simulink model "gm_UZ_EnDat_be4_segregation"  (R2023b)
settings: Solver=FixedStepAuto  StartTime=0  StopTime=0.000505  RelTol=1e-3
model workspace (MAT data in the model file):
  Select = 0
libraries: hdlsllib x74, simulink x21, hdlmdlgenlib x4, simulink_extras x1
(part 3 of 5)

== system gm_UZ_EnDat_be4_segregation/UZ_ENDAT/5timestorage/Compare To Constant ==
  u : Inport  OutDataTypeStr=fixdt(0,8,0,'DataTypeOverride', 'Off')  SampleTime=1e-08
  Compare : RelationalOperator  Operator===  OutDataTypeStr=boolean
  Constant : Constant  DisableCoverage=on  Value=const  OutDataTypeStr=Inherit: Inherit via back propagation  SampleTime=-1
  y : Outport  SampleTime=1e-08
  wires:
  u/1 -> Compare/1
  Compare/1 -> y/1
  Constant/1 -> Compare/2

== system gm_UZ_EnDat_be4_segregation/UZ_ENDAT/5timestorage/Compare To Constant1 ==
  u : Inport  OutDataTypeStr=fixdt(0,8,0,'DataTypeOverride', 'Off')  SampleTime=1e-08
  Compare : RelationalOperator  Operator===  OutDataTypeStr=boolean
  Constant : Constant  DisableCoverage=on  Value=const  OutDataTypeStr=Inherit: Inherit via back propagation  SampleTime=-1
  y : Outport  SampleTime=1e-08
  wires:
  u/1 -> Compare/1
  Compare/1 -> y/1
  Constant/1 -> Compare/2

== system gm_UZ_EnDat_be4_segregation/UZ_ENDAT/5timestorage/Compare To Constant2 ==
  u : Inport  OutDataTypeStr=fixdt(0,8,0,'DataTypeOverride', 'Off')  SampleTime=1e-08
  Compare : RelationalOperator  Operator===  OutDataTypeStr=boolean
  Constant : Constant  DisableCoverage=on  Value=const  OutDataTypeStr=Inherit: Inherit via back propagation  SampleTime=-1
  y : Outport  SampleTime=1e-08
  wires:
  u/1 -> Compare/1
  Compare/1 -> y/1
  Constant/1 -> Compare/2

== system gm_UZ_EnDat_be4_segregation/UZ_ENDAT/5timestorage/Compare To Constant3 ==
  u : Inport  OutDataTypeStr=fixdt(0,8,0,'DataTypeOverride', 'Off')  SampleTime=1e-08
  Compare : RelationalOperator  Operator===  OutDataTypeStr=boolean
  Constant : Constant  DisableCoverage=on  Value=const  OutDataTypeStr=Inherit: Inherit via back propagation  SampleTime=-1
  y : Outport  SampleTime=1e-08
  wires:
  u/1 -> Compare/1
  Compare/1 -> y/1
  Constant/1 -> Compare/2

== system gm_UZ_EnDat_be4_segregation/UZ_ENDAT/5timestorage/Compare To Constant4 ==
  u : Inport  OutDataTypeStr=fixdt(0,8,0,'DataTypeOverride', 'Off')  SampleTime=1e-08
  Compare : RelationalOperator  Operator===  OutDataTypeStr=boolean
  Constant : Constant  DisableCoverage=on  Value=const  OutDataTypeStr=Inherit: Inherit via back propagation  SampleTime=-1
  y : Outport  SampleTime=1e-08
  wires:
  u/1 -> Compare/1
  Compare/1 -> y/1
  Constant/1 -> Compare/2

== system gm_UZ_EnDat_be4_segregation/UZ_ENDAT/5timestorage/Storage20 ==
  Data : Inport  OutDataTypeStr=fixdt(0, 64, 0)  PortDimensions=1  SampleTime=1e-08
  Write : Inport  Port=2  OutDataTypeStr=boolean  PortDimensions=1  SampleTime=1e-08
  Compare To Zero : Subsystem  mask(Compare To Zero){relop===, OutDataTypeStr=boolean, ZeroCross=on}
      mask prompts: relop "Simulink:masks:Operator_MP"; OutDataTypeStr "Simulink:masks:OutputDataType_MP"; ZeroCross "Simulink:masks:EnableZerocrossingDetection_MP"
      mask help: Simulink:masks:CompareToZero_MD
      mask init:
      | OutDataTypeStr = 'boolean';
      | ZeroCross = 'on';
      | blkName = 'UZ_EnDat_be4_segregation/UZ_ENDAT/5timestorage/Storage20/Compare\nTo Zero';
      | relop = '==';
      | setValue = 'boolean';
      mask TypeOptions relop: == | ~= | < | <= | >= | >
      mask TypeOptions OutDataTypeStr: Simulink:masks:uint8 | Simulink:masks:boolean
      mask Callback ZeroCross: sl('zeroCrossEnable', gcbh);
      mask Display: disp([relop,' 0'])
  Logical Operator : Logic  Operator=NOT  Inputs=1  AllPortsSameDT=off  OutDataTypeStr=boolean  SampleTime=1e-08
  Logical Operator1 : Logic  Inputs=3  AllPortsSameDT=off  OutDataTypeStr=boolean  SampleTime=1e-08
  Logical Operator2 : Logic  Operator=NOT  Inputs=1  AllPortsSameDT=off  OutDataTypeStr=boolean  SampleTime=1e-08
  Relational Operator : RelationalOperator  Operator===  OutDataTypeStr=boolean  SampleTime=1e-08  InputSameDT=off
  Single Port RAM System : hdlsllib/HDL RAMs/Single Port RAM System  RAMType=Single port  AsyncRead=off  WriteOutputValue=Old data  RAMInitialValue=0  allowBusInputs=off  WritesHaveOutput=on  NumReads=0  NumWrites=1  SimulateUsing=Code generation
  adress : Constant  Value=20  OutDataTypeStr=uint8  SampleTime=1e-08
  t : Constant  Value=double(0)  OutDataTypeStr=boolean  SampleTime=1e-08
  out : Outport  SampleTime=1e-08
  wrok : Outport  Port=2  OutDataTypeStr=boolean  SampleTime=1e-08
  wires:
  Data/1 -> Compare To Zero/1(u), Relational Operator/2, Single Port RAM System/1
  Write/1 -> Logical Operator1/1
  Compare To Zero/1(y) -> Logical Operator2/1
  Logical Operator2/1 -> Logical Operator1/3
  t/1 -> wrok/1
  adress/1 -> Single Port RAM System/2
  Single Port RAM System/1 -> Relational Operator/1, out/1
  Relational Operator/1 -> Logical Operator/1
  Logical Operator/1 -> Logical Operator1/2
  Logical Operator1/1 -> Single Port RAM System/3

== system gm_UZ_EnDat_be4_segregation/UZ_ENDAT/5timestorage/Storage21 ==
  Data : Inport  OutDataTypeStr=fixdt(0, 64, 0)  PortDimensions=1  SampleTime=1e-08
  Write : Inport  Port=2  OutDataTypeStr=boolean  PortDimensions=1  SampleTime=1e-08
  Compare To Zero : Subsystem  mask(Compare To Zero){relop===, OutDataTypeStr=boolean, ZeroCross=on}
      mask prompts: relop "Simulink:masks:Operator_MP"; OutDataTypeStr "Simulink:masks:OutputDataType_MP"; ZeroCross "Simulink:masks:EnableZerocrossingDetection_MP"
      mask help: Simulink:masks:CompareToZero_MD
      mask init:
      | OutDataTypeStr = 'boolean';
      | ZeroCross = 'on';
      | blkName = 'UZ_EnDat_be4_segregation/UZ_ENDAT/5timestorage/Storage21/Compare\nTo Zero';
      | relop = '==';
      | setValue = 'boolean';
      mask TypeOptions relop: == | ~= | < | <= | >= | >
      mask TypeOptions OutDataTypeStr: Simulink:masks:uint8 | Simulink:masks:boolean
      mask Callback ZeroCross: sl('zeroCrossEnable', gcbh);
      mask Display: disp([relop,' 0'])
  Logical Operator : Logic  Operator=NOT  Inputs=1  AllPortsSameDT=off  OutDataTypeStr=boolean  SampleTime=1e-08
  Logical Operator1 : Logic  Inputs=3  AllPortsSameDT=off  OutDataTypeStr=boolean  SampleTime=1e-08
  Logical Operator2 : Logic  Operator=NOT  Inputs=1  AllPortsSameDT=off  OutDataTypeStr=boolean  SampleTime=1e-08
  Relational Operator : RelationalOperator  Operator===  OutDataTypeStr=boolean  SampleTime=1e-08  InputSameDT=off
  Single Port RAM System : hdlsllib/HDL RAMs/Single Port RAM System  RAMType=Single port  AsyncRead=off  WriteOutputValue=Old data  RAMInitialValue=0  allowBusInputs=off  WritesHaveOutput=on  NumReads=0  NumWrites=1  SimulateUsing=Code generation
  adress : Constant  Value=21  OutDataTypeStr=uint8  SampleTime=1e-08
  t : Constant  Value=double(0)  OutDataTypeStr=boolean  SampleTime=1e-08
  out : Outport  SampleTime=1e-08
  wrok : Outport  Port=2  OutDataTypeStr=boolean  SampleTime=1e-08
  wires:
  Data/1 -> Compare To Zero/1(u), Relational Operator/2, Single Port RAM System/1
  Write/1 -> Logical Operator1/1
  Compare To Zero/1(y) -> Logical Operator2/1
  Logical Operator2/1 -> Logical Operator1/3
  t/1 -> wrok/1
  adress/1 -> Single Port RAM System/2
  Single Port RAM System/1 -> Relational Operator/1, out/1
  Relational Operator/1 -> Logical Operator/1
  Logical Operator/1 -> Logical Operator1/2
  Logical Operator1/1 -> Single Port RAM System/3

== system gm_UZ_EnDat_be4_segregation/UZ_ENDAT/5timestorage/Storage22 ==
  Data : Inport  OutDataTypeStr=fixdt(0, 64, 0)  PortDimensions=1  SampleTime=1e-08
  Write : Inport  Port=2  OutDataTypeStr=boolean  PortDimensions=1  SampleTime=1e-08
  Compare To Zero : Subsystem  mask(Compare To Zero){relop===, OutDataTypeStr=boolean, ZeroCross=on}
      mask prompts: relop "Simulink:masks:Operator_MP"; OutDataTypeStr "Simulink:masks:OutputDataType_MP"; ZeroCross "Simulink:masks:EnableZerocrossingDetection_MP"
      mask help: Simulink:masks:CompareToZero_MD
      mask init:
      | OutDataTypeStr = 'boolean';
      | ZeroCross = 'on';
      | blkName = 'UZ_EnDat_be4_segregation/UZ_ENDAT/5timestorage/Storage22/Compare\nTo Zero';
      | relop = '==';
      | setValue = 'boolean';
      mask TypeOptions relop: == | ~= | < | <= | >= | >
      mask TypeOptions OutDataTypeStr: Simulink:masks:uint8 | Simulink:masks:boolean
      mask Callback ZeroCross: sl('zeroCrossEnable', gcbh);
      mask Display: disp([relop,' 0'])
  Logical Operator : Logic  Operator=NOT  Inputs=1  AllPortsSameDT=off  OutDataTypeStr=boolean  SampleTime=1e-08
  Logical Operator1 : Logic  Inputs=3  AllPortsSameDT=off  OutDataTypeStr=boolean  SampleTime=1e-08
  Logical Operator2 : Logic  Operator=NOT  Inputs=1  AllPortsSameDT=off  OutDataTypeStr=boolean  SampleTime=1e-08
  Relational Operator : RelationalOperator  Operator===  OutDataTypeStr=boolean  SampleTime=1e-08  InputSameDT=off
  Single Port RAM System : hdlsllib/HDL RAMs/Single Port RAM System  RAMType=Single port  AsyncRead=off  WriteOutputValue=Old data  RAMInitialValue=0  allowBusInputs=off  WritesHaveOutput=on  NumReads=0  NumWrites=1  SimulateUsing=Code generation
  adress : Constant  Value=22  OutDataTypeStr=uint8  SampleTime=1e-08
  t : Constant  Value=double(0)  OutDataTypeStr=boolean  SampleTime=1e-08
  out : Outport  SampleTime=1e-08
  wrok : Outport  Port=2  OutDataTypeStr=boolean  SampleTime=1e-08
  wires:
  Data/1 -> Compare To Zero/1(u), Relational Operator/2, Single Port RAM System/1
  Write/1 -> Logical Operator1/1
  Compare To Zero/1(y) -> Logical Operator2/1
  Logical Operator2/1 -> Logical Operator1/3
  t/1 -> wrok/1
  adress/1 -> Single Port RAM System/2
  Single Port RAM System/1 -> Relational Operator/1, out/1
  Relational Operator/1 -> Logical Operator/1
  Logical Operator/1 -> Logical Operator1/2
  Logical Operator1/1 -> Single Port RAM System/3

== system gm_UZ_EnDat_be4_segregation/UZ_ENDAT/5timestorage/Storage23 ==
  Data : Inport  OutDataTypeStr=fixdt(0, 64, 0)  PortDimensions=1  SampleTime=1e-08
  Write : Inport  Port=2  OutDataTypeStr=boolean  PortDimensions=1  SampleTime=1e-08
  Compare To Zero : Subsystem  mask(Compare To Zero){relop===, OutDataTypeStr=boolean, ZeroCross=on}
      mask prompts: relop "Simulink:masks:Operator_MP"; OutDataTypeStr "Simulink:masks:OutputDataType_MP"; ZeroCross "Simulink:masks:EnableZerocrossingDetection_MP"
      mask help: Simulink:masks:CompareToZero_MD
      mask init:
      | OutDataTypeStr = 'boolean';
      | ZeroCross = 'on';
      | blkName = 'UZ_EnDat_be4_segregation/UZ_ENDAT/5timestorage/Storage23/Compare\nTo Zero';
      | relop = '==';
      | setValue = 'boolean';
      mask TypeOptions relop: == | ~= | < | <= | >= | >
      mask TypeOptions OutDataTypeStr: Simulink:masks:uint8 | Simulink:masks:boolean
      mask Callback ZeroCross: sl('zeroCrossEnable', gcbh);
      mask Display: disp([relop,' 0'])
  Logical Operator : Logic  Operator=NOT  Inputs=1  AllPortsSameDT=off  OutDataTypeStr=boolean  SampleTime=1e-08
  Logical Operator1 : Logic  Inputs=3  AllPortsSameDT=off  OutDataTypeStr=boolean  SampleTime=1e-08
  Logical Operator2 : Logic  Operator=NOT  Inputs=1  AllPortsSameDT=off  OutDataTypeStr=boolean  SampleTime=1e-08
  Relational Operator : RelationalOperator  Operator===  OutDataTypeStr=boolean  SampleTime=1e-08  InputSameDT=off
  Single Port RAM System : hdlsllib/HDL RAMs/Single Port RAM System  RAMType=Single port  AsyncRead=off  WriteOutputValue=Old data  RAMInitialValue=0  allowBusInputs=off  WritesHaveOutput=on  NumReads=0  NumWrites=1  SimulateUsing=Code generation
  adress : Constant  Value=23  OutDataTypeStr=uint8  SampleTime=1e-08
  t : Constant  Value=double(0)  OutDataTypeStr=boolean  SampleTime=1e-08
  out : Outport  SampleTime=1e-08
  wrok : Outport  Port=2  OutDataTypeStr=boolean  SampleTime=1e-08
  wires:
  Data/1 -> Compare To Zero/1(u), Relational Operator/2, Single Port RAM System/1
  Write/1 -> Logical Operator1/1
  Compare To Zero/1(y) -> Logical Operator2/1
  Logical Operator2/1 -> Logical Operator1/3
  t/1 -> wrok/1
  adress/1 -> Single Port RAM System/2
  Single Port RAM System/1 -> Relational Operator/1, out/1
  Relational Operator/1 -> Logical Operator/1
  Logical Operator/1 -> Logical Operator1/2
  Logical Operator1/1 -> Single Port RAM System/3

== system gm_UZ_EnDat_be4_segregation/UZ_ENDAT/5timestorage/Storage24 ==
  Data : Inport  OutDataTypeStr=fixdt(0, 64, 0)  PortDimensions=1  SampleTime=1e-08
  Write : Inport  Port=2  OutDataTypeStr=boolean  PortDimensions=1  SampleTime=1e-08
  Compare To Zero : Subsystem  mask(Compare To Zero){relop===, OutDataTypeStr=boolean, ZeroCross=on}
      mask prompts: relop "Simulink:masks:Operator_MP"; OutDataTypeStr "Simulink:masks:OutputDataType_MP"; ZeroCross "Simulink:masks:EnableZerocrossingDetection_MP"
      mask help: Simulink:masks:CompareToZero_MD
      mask init:
      | OutDataTypeStr = 'boolean';
      | ZeroCross = 'on';
      | blkName = 'UZ_EnDat_be4_segregation/UZ_ENDAT/5timestorage/Storage24/Compare\nTo Zero';
      | relop = '==';
      | setValue = 'boolean';
      mask TypeOptions relop: == | ~= | < | <= | >= | >
      mask TypeOptions OutDataTypeStr: Simulink:masks:uint8 | Simulink:masks:boolean
      mask Callback ZeroCross: sl('zeroCrossEnable', gcbh);
      mask Display: disp([relop,' 0'])
  Logical Operator : Logic  Operator=NOT  Inputs=1  AllPortsSameDT=off  OutDataTypeStr=boolean  SampleTime=1e-08
  Logical Operator1 : Logic  Inputs=3  AllPortsSameDT=off  OutDataTypeStr=boolean  SampleTime=1e-08
  Logical Operator2 : Logic  Operator=NOT  Inputs=1  AllPortsSameDT=off  OutDataTypeStr=boolean  SampleTime=1e-08
  Relational Operator : RelationalOperator  Operator===  OutDataTypeStr=boolean  SampleTime=1e-08  InputSameDT=off
  Single Port RAM System : hdlsllib/HDL RAMs/Single Port RAM System  RAMType=Single port  AsyncRead=off  WriteOutputValue=Old data  RAMInitialValue=0  allowBusInputs=off  WritesHaveOutput=on  NumReads=0  NumWrites=1  SimulateUsing=Code generation
  adress : Constant  Value=24  OutDataTypeStr=uint8  SampleTime=1e-08
  t : Constant  Value=double(0)  OutDataTypeStr=boolean  SampleTime=1e-08
  out : Outport  SampleTime=1e-08
  wrok : Outport  Port=2  OutDataTypeStr=boolean  SampleTime=1e-08
  wires:
  Data/1 -> Compare To Zero/1(u), Relational Operator/2, Single Port RAM System/1
  Write/1 -> Logical Operator1/1
  Compare To Zero/1(y) -> Logical Operator2/1
  Logical Operator2/1 -> Logical Operator1/3
  t/1 -> wrok/1
  adress/1 -> Single Port RAM System/2
  Single Port RAM System/1 -> Relational Operator/1, out/1
  Relational Operator/1 -> Logical Operator/1
  Logical Operator/1 -> Logical Operator1/2
  Logical Operator1/1 -> Single Port RAM System/3

== system gm_UZ_EnDat_be4_segregation/UZ_ENDAT/5timestorage/Triggered Subsystem ==
  Trigger : Inport  OutDataTypeStr=boolean  SampleTime=1e-08
  Counter Limited : Subsystem  mask(Counter Limited){uplimit=double(4), tsamp=double(-1)}
      mask prompts: uplimit "Simulink:masks:UpperLimit_MP"; tsamp "Simulink:masks:SampleTime_MP"
      mask help: Simulink:masks:CounterLimited_MD
  Trigger_delay : Delay  DelayLength=double(1)  InitialCondition=0
  Trigger_delay_Initial_Val : Constant  OutDataTypeStr=boolean  SampleTime=1e-08
  Trigger_delay_ctrl_const : Constant  OutDataTypeStr=boolean  SampleTime=1e-08
  Trigger_delay_ctrl_delay : Delay  DelayLength=double(1)  InitialCondition=0
  Trigger_delay_switch : Switch  Criteria=u2 ~= 0  Threshold=double(0)  OutDataTypeStr=boolean  SampleTime=1e-08  SaturateOnIntegerOverflow=off  InputSameDT=off
  Trigger_delayed_inverted_and_Trigger : Logic  AllPortsSameDT=off  OutDataTypeStr=boolean  SampleTime=1e-08
  delayMatch : Delay  DelayLength=double(2)  InitialCondition=0
  not_Trigger_delayed : Logic  Operator=NOT  Inputs=1  AllPortsSameDT=off  OutDataTypeStr=boolean  SampleTime=1e-08
  Out1 : Outport  SampleTime=1e-08  InitialOutput=0
  wires:
  Trigger/1 -> Trigger_delayed_inverted_and_Trigger/2, Trigger_delay/1
  Counter Limited/1(y) -> Out1/1
  Trigger_delay_switch/1 -> not_Trigger_delayed/1
  not_Trigger_delayed/1 -> Trigger_delayed_inverted_and_Trigger/1
  Trigger_delayed_inverted_and_Trigger/1 -> Counter Limited/1(Trigger_emulated)
  Trigger_delay/1 -> Trigger_delay_switch/1
  Trigger_delay_Initial_Val/1 -> Trigger_delay_switch/3
  Trigger_delay_ctrl_const/1 -> Trigger_delay_ctrl_delay/1
  delayMatch/1 -> Trigger_delay_switch/2
  Trigger_delay_ctrl_delay/1 -> delayMatch/1

== system gm_UZ_EnDat_be4_segregation/UZ_ENDAT/CLKCNTER_ACT/Positional_Counter ==
  valueout : Inport  OutDataTypeStr=uint32  PortDimensions=1  SampleTime=1e-08
  Trigger : Inport  Port=2  OutDataTypeStr=boolean  SampleTime=1e-08
  Increment Stored Integer : Subsystem  mask(Stored Integer Value Increment){}
      mask help: Simulink:masks:StoredIntegerValueIncrement_MD
      mask Display: disp('Q++')
  Increment Stored Integer_out1bypassMux : MultiPortSwitch  DataPortOrder=Zero-based contiguous  Inputs=2  zeroidx=on  OutDataTypeStr=uint32  SampleTime=1e-08  SaturateOnIntegerOverflow=off  InputSameDT=off
  Trigger_delay : Delay  DelayLength=double(1)  InitialCondition=0
  Trigger_delayed_inverted_and_Trigger : Logic  AllPortsSameDT=off  OutDataTypeStr=boolean  SampleTime=1e-08
  not_Trigger_delayed : Logic  Operator=NOT  Inputs=1  AllPortsSameDT=off  OutDataTypeStr=boolean  SampleTime=1e-08
  out0_bypass : UnitDelay  InitialCondition="fi(0,0,32,0,\"hex\",\"00000000\")"  SampleTime=1e-08
  divider : Outport  SampleTime=1e-08  InitialOutput=0
  wires:
  Increment Stored Integer/1(y) -> Increment Stored Integer_out1bypassMux/3
  out0_bypass/1 -> Increment Stored Integer_out1bypassMux/2
  Trigger_delayed_inverted_and_Trigger/1 -> Increment Stored Integer_out1bypassMux/1
  not_Trigger_delayed/1 -> Trigger_delayed_inverted_and_Trigger/1
  Trigger_delay/1 -> not_Trigger_delayed/1
  Increment Stored Integer_out1bypassMux/1 -> out0_bypass/1, divider/1
  valueout/1 -> Increment Stored Integer/1(u)
  Trigger/1 -> Trigger_delay/1, Trigger_delayed_inverted_and_Trigger/2

== system gm_UZ_EnDat_be4_segregation/UZ_ENDAT/CLKCNTER_ACT/SetZero32 ==
  valin : Inport  OutDataTypeStr=uint32  PortDimensions=1  SampleTime=1e-08
  setzero : Inport  Port=2  OutDataTypeStr=boolean  PortDimensions=1  SampleTime=1e-08
  Trigger : Inport  Port=3  OutDataTypeStr=boolean  SampleTime=1e-08
  Constant1 : Constant  OutDataTypeStr=fixdt(0, 1, 0)  SampleTime=1e-08
  Constant2 : Constant  Value=0  OutDataTypeStr=fixdt(0, 1, 0)  SampleTime=1e-08
  Index Vector1 : MultiPortSwitch  DataPortOrder=Zero-based contiguous  Inputs=2  DiagnosticForDefault=None  zeroidx=on  OutDataTypeStr=fixdt(0, 1, 0)  SampleTime=1e-08  SaturateOnIntegerOverflow=off  InputSameDT=off
  Product : Product  Inputs=**  OutDataTypeStr=uint32  SaturateOnIntegerOverflow=on  SampleTime=1e-08
  Product_out1bypassMux : MultiPortSwitch  DataPortOrder=Zero-based contiguous  Inputs=2  zeroidx=on  OutDataTypeStr=uint32  SampleTime=1e-08  SaturateOnIntegerOverflow=off  InputSameDT=off
  Trigger_delay : Delay  DelayLength=double(1)  InitialCondition=0
  Trigger_delay_Initial_Val : Constant  OutDataTypeStr=boolean  SampleTime=1e-08
  Trigger_delay_ctrl_const : Constant  OutDataTypeStr=boolean  SampleTime=1e-08
  Trigger_delay_ctrl_delay : Delay  DelayLength=double(1)  InitialCondition=0
  Trigger_delay_switch : Switch  Criteria=u2 ~= 0  Threshold=double(0)  OutDataTypeStr=boolean  SampleTime=1e-08  SaturateOnIntegerOverflow=off  InputSameDT=off
  Trigger_delayed_inverted_and_Trigger : Logic  AllPortsSameDT=off  OutDataTypeStr=boolean  SampleTime=1e-08
  delayMatch{,1..5} (6 alike) : Delay  DelayLength=double(2)  InitialCondition=0
  not_Trigger_delayed : Logic  Operator=NOT  Inputs=1  AllPortsSameDT=off  OutDataTypeStr=boolean  SampleTime=1e-08
  out0_bypass : UnitDelay  InitialCondition=double(0)  SampleTime=1e-08
  out0_bypass_Initial_Val : Constant  OutDataTypeStr=uint32  SampleTime=1e-08
  out0_bypass_ctrl_const : Constant  OutDataTypeStr=boolean  SampleTime=1e-08
  out0_bypass_ctrl_delay : Delay  DelayLength=double(1)  InitialCondition=0
  out0_bypass_switch : Switch  Criteria=u2 ~= 0  Threshold=double(0)  OutDataTypeStr=uint32  SampleTime=1e-08  SaturateOnIntegerOverflow=off  InputSameDT=off
  valueout : Outport  SampleTime=1e-08  InitialOutput=0  VectorParamsAs1DForOutWhenUnconnected=off
  wires:
  Trigger/1 -> Trigger_delayed_inverted_and_Trigger/2, Trigger_delay/1
  valin/1 -> Product/2
  setzero/1 -> Index Vector1/1
  Trigger_delay_switch/1 -> not_Trigger_delayed/1
  not_Trigger_delayed/1 -> Trigger_delayed_inverted_and_Trigger/1
  Trigger_delay/1 -> Trigger_delay_switch/1
  delayMatch1/1 -> Trigger_delay_switch/3
  delayMatch/1 -> Trigger_delay_switch/2
  Index Vector1/1 -> Product/1
  delayMatch2/1 -> Index Vector1/2
  delayMatch3/1 -> Index Vector1/3
  Trigger_delay_ctrl_delay/1 -> delayMatch/1
  Trigger_delay_Initial_Val/1 -> delayMatch1/1
  Constant1/1 -> delayMatch2/1
  Constant2/1 -> delayMatch3/1
  out0_bypass_ctrl_delay/1 -> delayMatch4/1
  out0_bypass_Initial_Val/1 -> delayMatch5/1
  Product_out1bypassMux/1 -> out0_bypass/1, valueout/1
  out0_bypass/1 -> out0_bypass_switch/1
  delayMatch4/1 -> out0_bypass_switch/2
  delayMatch5/1 -> out0_bypass_switch/3
  Trigger_delayed_inverted_and_Trigger/1 -> Product_out1bypassMux/1
  Product/1 -> Product_out1bypassMux/3
  out0_bypass_switch/1 -> Product_out1bypassMux/2
  out0_bypass_ctrl_const/1 -> out0_bypass_ctrl_delay/1
  Trigger_delay_ctrl_const/1 -> Trigger_delay_ctrl_delay/1

== system gm_UZ_EnDat_be4_segregation/UZ_ENDAT/CLKCNTER_RAMPUP/Positional_Counter ==
  valueout : Inport  OutDataTypeStr=uint32  PortDimensions=1  SampleTime=1e-08
  Trigger : Inport  Port=2  OutDataTypeStr=boolean  SampleTime=1e-08
  Increment Stored Integer : Subsystem  mask(Stored Integer Value Increment){}
      mask help: Simulink:masks:StoredIntegerValueIncrement_MD
      mask Display: disp('Q++')
  Increment Stored Integer_out1bypassMux : MultiPortSwitch  DataPortOrder=Zero-based contiguous  Inputs=2  zeroidx=on  OutDataTypeStr=uint32  SampleTime=1e-08  SaturateOnIntegerOverflow=off  InputSameDT=off
  Trigger_delay : Delay  DelayLength=double(1)  InitialCondition=0
  Trigger_delayed_inverted_and_Trigger : Logic  AllPortsSameDT=off  OutDataTypeStr=boolean  SampleTime=1e-08
  not_Trigger_delayed : Logic  Operator=NOT  Inputs=1  AllPortsSameDT=off  OutDataTypeStr=boolean  SampleTime=1e-08
  out0_bypass : UnitDelay  InitialCondition="fi(0,0,32,0,\"hex\",\"00000000\")"  SampleTime=1e-08
  divider : Outport  SampleTime=1e-08  InitialOutput=0
  wires:
  Increment Stored Integer/1(y) -> Increment Stored Integer_out1bypassMux/3
  out0_bypass/1 -> Increment Stored Integer_out1bypassMux/2
  Trigger_delayed_inverted_and_Trigger/1 -> Increment Stored Integer_out1bypassMux/1
  not_Trigger_delayed/1 -> Trigger_delayed_inverted_and_Trigger/1
  Trigger_delay/1 -> not_Trigger_delayed/1
  Increment Stored Integer_out1bypassMux/1 -> out0_bypass/1, divider/1
  valueout/1 -> Increment Stored Integer/1(u)
  Trigger/1 -> Trigger_delay/1, Trigger_delayed_inverted_and_Trigger/2

== system gm_UZ_EnDat_be4_segregation/UZ_ENDAT/CLKCNTER_RAMPUP/SetZero32 ==
  valin : Inport  OutDataTypeStr=uint32  PortDimensions=1  SampleTime=1e-08
  setzero : Inport  Port=2  OutDataTypeStr=boolean  PortDimensions=1  SampleTime=1e-08
  Trigger : Inport  Port=3  OutDataTypeStr=boolean  SampleTime=1e-08
  Constant1 : Constant  OutDataTypeStr=fixdt(0, 1, 0)  SampleTime=1e-08
  Constant2 : Constant  Value=0  OutDataTypeStr=fixdt(0, 1, 0)  SampleTime=1e-08
  Index Vector1 : MultiPortSwitch  DataPortOrder=Zero-based contiguous  Inputs=2  DiagnosticForDefault=None  zeroidx=on  OutDataTypeStr=fixdt(0, 1, 0)  SampleTime=1e-08  SaturateOnIntegerOverflow=off  InputSameDT=off
  Product : Product  Inputs=**  OutDataTypeStr=uint32  SaturateOnIntegerOverflow=on  SampleTime=1e-08
  Product_out1bypassMux : MultiPortSwitch  DataPortOrder=Zero-based contiguous  Inputs=2  zeroidx=on  OutDataTypeStr=uint32  SampleTime=1e-08  SaturateOnIntegerOverflow=off  InputSameDT=off
  Trigger_delay : Delay  DelayLength=double(1)  InitialCondition=0
  Trigger_delay_Initial_Val : Constant  OutDataTypeStr=boolean  SampleTime=1e-08
  Trigger_delay_ctrl_const : Constant  OutDataTypeStr=boolean  SampleTime=1e-08
  Trigger_delay_ctrl_delay : Delay  DelayLength=double(1)  InitialCondition=0
  Trigger_delay_switch : Switch  Criteria=u2 ~= 0  Threshold=double(0)  OutDataTypeStr=boolean  SampleTime=1e-08  SaturateOnIntegerOverflow=off  InputSameDT=off
  Trigger_delayed_inverted_and_Trigger : Logic  AllPortsSameDT=off  OutDataTypeStr=boolean  SampleTime=1e-08
  not_Trigger_delayed : Logic  Operator=NOT  Inputs=1  AllPortsSameDT=off  OutDataTypeStr=boolean  SampleTime=1e-08
  out0_bypass : UnitDelay  InitialCondition=double(0)  SampleTime=1e-08
  out0_bypass_Initial_Val : Constant  OutDataTypeStr=uint32  SampleTime=1e-08
  out0_bypass_ctrl_const : Constant  OutDataTypeStr=boolean  SampleTime=1e-08
  out0_bypass_ctrl_delay : Delay  DelayLength=double(1)  InitialCondition=0
  out0_bypass_switch : Switch  Criteria=u2 ~= 0  Threshold=double(0)  OutDataTypeStr=uint32  SampleTime=1e-08  SaturateOnIntegerOverflow=off  InputSameDT=off
  valueout : Outport  SampleTime=1e-08  InitialOutput=0  VectorParamsAs1DForOutWhenUnconnected=off
  wires:
  Trigger/1 -> Trigger_delayed_inverted_and_Trigger/2, Trigger_delay/1
  valin/1 -> Product/2
  setzero/1 -> Index Vector1/1
  Product_out1bypassMux/1 -> valueout/1, out0_bypass/1
  Trigger_delay_switch/1 -> not_Trigger_delayed/1
  not_Trigger_delayed/1 -> Trigger_delayed_inverted_and_Trigger/1
  Trigger_delay/1 -> Trigger_delay_switch/1
  Trigger_delay_Initial_Val/1 -> Trigger_delay_switch/3
  Trigger_delay_ctrl_delay/1 -> Trigger_delay_switch/2
  Index Vector1/1 -> Product/1
  Constant1/1 -> Index Vector1/2
  Constant2/1 -> Index Vector1/3
  out0_bypass/1 -> out0_bypass_switch/1
  out0_bypass_ctrl_delay/1 -> out0_bypass_switch/2
  out0_bypass_Initial_Val/1 -> out0_bypass_switch/3
  Trigger_delayed_inverted_and_Trigger/1 -> Product_out1bypassMux/1
  Product/1 -> Product_out1bypassMux/3
  out0_bypass_switch/1 -> Product_out1bypassMux/2
  out0_bypass_ctrl_const/1 -> out0_bypass_ctrl_delay/1
  Trigger_delay_ctrl_const/1 -> Trigger_delay_ctrl_delay/1

== system gm_UZ_EnDat_be4_segregation/UZ_ENDAT/CLKDIV1/Triggered Subsystem ==
  D : Inport  OutDataTypeStr=boolean  PortDimensions=1  SampleTime=1e-08
  Trigger : Inport  Port=2  OutDataTypeStr=boolean  SampleTime=1e-08
  DbypassMux : MultiPortSwitch  DataPortOrder=Zero-based contiguous  Inputs=2  zeroidx=on  SampleTime=1e-08  SaturateOnIntegerOverflow=off  InputSameDT=off
  Trigger_delay : Delay  DelayLength=double(1)  InitialCondition=0
  Trigger_delay_Initial_Val : Constant  OutDataTypeStr=boolean  SampleTime=1e-08
  Trigger_delay_ctrl_const : Constant  OutDataTypeStr=boolean  SampleTime=1e-08
  Trigger_delay_ctrl_delay : Delay  DelayLength=double(1)  InitialCondition=0
  Trigger_delay_switch : Switch  Criteria=u2 ~= 0  Threshold=double(0)  OutDataTypeStr=boolean  SampleTime=1e-08  SaturateOnIntegerOverflow=off  InputSameDT=off
  Trigger_delayed_inverted_and_Trigger : Logic  AllPortsSameDT=off  OutDataTypeStr=boolean  SampleTime=1e-08
  not_Trigger_delayed : Logic  Operator=NOT  Inputs=1  AllPortsSameDT=off  OutDataTypeStr=boolean  SampleTime=1e-08
  out0_bypass : UnitDelay  SampleTime=1e-08
  Q : Outport  SampleTime=1e-08  InitialOutput=0
  wires:
  Trigger/1 -> Trigger_delayed_inverted_and_Trigger/2, Trigger_delay/1
  DbypassMux/1 -> Q/1, out0_bypass/1
  Trigger_delay_switch/1 -> not_Trigger_delayed/1
  not_Trigger_delayed/1 -> Trigger_delayed_inverted_and_Trigger/1
  Trigger_delay/1 -> Trigger_delay_switch/1
  Trigger_delay_Initial_Val/1 -> Trigger_delay_switch/3
  Trigger_delay_ctrl_delay/1 -> Trigger_delay_switch/2
  Trigger_delayed_inverted_and_Trigger/1 -> DbypassMux/1
  out0_bypass/1 -> DbypassMux/2
  D/1 -> DbypassMux/3
  Trigger_delay_ctrl_const/1 -> Trigger_delay_ctrl_delay/1

== system gm_UZ_EnDat_be4_segregation/UZ_ENDAT/CLKDIV3/Triggered Subsystem ==
  D : Inport  OutDataTypeStr=boolean  PortDimensions=1  SampleTime=1e-08
  Trigger : Inport  Port=2  OutDataTypeStr=boolean  SampleTime=1e-08
  DbypassMux : MultiPortSwitch  DataPortOrder=Zero-based contiguous  Inputs=2  zeroidx=on  SampleTime=1e-08  SaturateOnIntegerOverflow=off  InputSameDT=off
  Trigger_delay : Delay  DelayLength=double(1)  InitialCondition=0
  Trigger_delay_Initial_Val : Constant  OutDataTypeStr=boolean  SampleTime=1e-08
  Trigger_delay_ctrl_const : Constant  OutDataTypeStr=boolean  SampleTime=1e-08
  Trigger_delay_ctrl_delay : Delay  DelayLength=double(1)  InitialCondition=0
  Trigger_delay_switch : Switch  Criteria=u2 ~= 0  Threshold=double(0)  OutDataTypeStr=boolean  SampleTime=1e-08  SaturateOnIntegerOverflow=off  InputSameDT=off
  Trigger_delayed_inverted_and_Trigger : Logic  AllPortsSameDT=off  OutDataTypeStr=boolean  SampleTime=1e-08
  not_Trigger_delayed : Logic  Operator=NOT  Inputs=1  AllPortsSameDT=off  OutDataTypeStr=boolean  SampleTime=1e-08
  out0_bypass : UnitDelay  SampleTime=1e-08
  Q : Outport  SampleTime=1e-08  InitialOutput=0
  wires:
  Trigger_delay_ctrl_const/1 -> Trigger_delay_ctrl_delay/1
  D/1 -> DbypassMux/3
  out0_bypass/1 -> DbypassMux/2
  Trigger_delayed_inverted_and_Trigger/1 -> DbypassMux/1
  Trigger_delay_ctrl_delay/1 -> Trigger_delay_switch/2
  Trigger_delay_Initial_Val/1 -> Trigger_delay_switch/3
  Trigger_delay/1 -> Trigger_delay_switch/1
  not_Trigger_delayed/1 -> Trigger_delayed_inverted_and_Trigger/1
  Trigger_delay_switch/1 -> not_Trigger_delayed/1
  DbypassMux/1 -> out0_bypass/1, Q/1
  Trigger/1 -> Trigger_delay/1, Trigger_delayed_inverted_and_Trigger/2

== system gm_UZ_EnDat_be4_segregation/UZ_ENDAT/CLKDIV4/Triggered Subsystem ==
  D : Inport  OutDataTypeStr=boolean  PortDimensions=1  SampleTime=1e-08
  Trigger : Inport  Port=2  OutDataTypeStr=boolean  SampleTime=1e-08
  DbypassMux : MultiPortSwitch  DataPortOrder=Zero-based contiguous  Inputs=2  zeroidx=on  SampleTime=1e-08  SaturateOnIntegerOverflow=off  InputSameDT=off
  Trigger_delay : Delay  DelayLength=double(1)  InitialCondition=0
  Trigger_delay_Initial_Val : Constant  OutDataTypeStr=boolean  SampleTime=1e-08
  Trigger_delay_ctrl_const : Constant  OutDataTypeStr=boolean  SampleTime=1e-08
  Trigger_delay_ctrl_delay : Delay  DelayLength=double(1)  InitialCondition=0
  Trigger_delay_switch : Switch  Criteria=u2 ~= 0  Threshold=double(0)  OutDataTypeStr=boolean  SampleTime=1e-08  SaturateOnIntegerOverflow=off  InputSameDT=off
  Trigger_delayed_inverted_and_Trigger : Logic  AllPortsSameDT=off  OutDataTypeStr=boolean  SampleTime=1e-08
  not_Trigger_delayed : Logic  Operator=NOT  Inputs=1  AllPortsSameDT=off  OutDataTypeStr=boolean  SampleTime=1e-08
  out0_bypass : UnitDelay  SampleTime=1e-08
  Q : Outport  SampleTime=1e-08  InitialOutput=0
  wires:
  Trigger_delay_ctrl_const/1 -> Trigger_delay_ctrl_delay/1
  D/1 -> DbypassMux/3
  out0_bypass/1 -> DbypassMux/2
  Trigger_delayed_inverted_and_Trigger/1 -> DbypassMux/1
  Trigger_delay_ctrl_delay/1 -> Trigger_delay_switch/2
  Trigger_delay_Initial_Val/1 -> Trigger_delay_switch/3
  Trigger_delay/1 -> Trigger_delay_switch/1
  not_Trigger_delayed/1 -> Trigger_delayed_inverted_and_Trigger/1
  Trigger_delay_switch/1 -> not_Trigger_delayed/1
  DbypassMux/1 -> out0_bypass/1, Q/1
  Trigger/1 -> Trigger_delay/1, Trigger_delayed_inverted_and_Trigger/2

== system gm_UZ_EnDat_be4_segregation/UZ_ENDAT/CLKDIV5/Triggered Subsystem ==
  D : Inport  OutDataTypeStr=boolean  PortDimensions=1  SampleTime=1e-08
  Trigger : Inport  Port=2  OutDataTypeStr=boolean  SampleTime=1e-08
  DbypassMux : MultiPortSwitch  DataPortOrder=Zero-based contiguous  Inputs=2  zeroidx=on  SampleTime=1e-08  SaturateOnIntegerOverflow=off  InputSameDT=off
  Trigger_delay : Delay  DelayLength=double(1)  InitialCondition=0
  Trigger_delay_Initial_Val : Constant  OutDataTypeStr=boolean  SampleTime=1e-08
  Trigger_delay_ctrl_const : Constant  OutDataTypeStr=boolean  SampleTime=1e-08
  Trigger_delay_ctrl_delay : Delay  DelayLength=double(1)  InitialCondition=0
  Trigger_delay_switch : Switch  Criteria=u2 ~= 0  Threshold=double(0)  OutDataTypeStr=boolean  SampleTime=1e-08  SaturateOnIntegerOverflow=off  InputSameDT=off
  Trigger_delayed_inverted_and_Trigger : Logic  AllPortsSameDT=off  OutDataTypeStr=boolean  SampleTime=1e-08
  not_Trigger_delayed : Logic  Operator=NOT  Inputs=1  AllPortsSameDT=off  OutDataTypeStr=boolean  SampleTime=1e-08
  out0_bypass : UnitDelay  SampleTime=1e-08
  Q : Outport  SampleTime=1e-08  InitialOutput=0
  wires:
  Trigger_delay_ctrl_const/1 -> Trigger_delay_ctrl_delay/1
  D/1 -> DbypassMux/3
  out0_bypass/1 -> DbypassMux/2
  Trigger_delayed_inverted_and_Trigger/1 -> DbypassMux/1
  Trigger_delay_ctrl_delay/1 -> Trigger_delay_switch/2
  Trigger_delay_Initial_Val/1 -> Trigger_delay_switch/3
  Trigger_delay/1 -> Trigger_delay_switch/1
  not_Trigger_delayed/1 -> Trigger_delayed_inverted_and_Trigger/1
  Trigger_delay_switch/1 -> not_Trigger_delayed/1
  DbypassMux/1 -> out0_bypass/1, Q/1
  Trigger/1 -> Trigger_delay/1, Trigger_delayed_inverted_and_Trigger/2

== system gm_UZ_EnDat_be4_segregation/UZ_ENDAT/CLKDIV6/Triggered Subsystem ==
  D : Inport  OutDataTypeStr=boolean  PortDimensions=1  SampleTime=1e-08
  Trigger : Inport  Port=2  OutDataTypeStr=boolean  SampleTime=1e-08
  DbypassMux : MultiPortSwitch  DataPortOrder=Zero-based contiguous  Inputs=2  zeroidx=on  SampleTime=1e-08  SaturateOnIntegerOverflow=off  InputSameDT=off
  Trigger_delay : Delay  DelayLength=double(1)  InitialCondition=0
  Trigger_delay_Initial_Val : Constant  OutDataTypeStr=boolean  SampleTime=1e-08
  Trigger_delay_ctrl_const : Constant  OutDataTypeStr=boolean  SampleTime=1e-08
  Trigger_delay_ctrl_delay : Delay  DelayLength=double(1)  InitialCondition=0
  Trigger_delay_switch : Switch  Criteria=u2 ~= 0  Threshold=double(0)  OutDataTypeStr=boolean  SampleTime=1e-08  SaturateOnIntegerOverflow=off  InputSameDT=off
  Trigger_delayed_inverted_and_Trigger : Logic  AllPortsSameDT=off  OutDataTypeStr=boolean  SampleTime=1e-08
  not_Trigger_delayed : Logic  Operator=NOT  Inputs=1  AllPortsSameDT=off  OutDataTypeStr=boolean  SampleTime=1e-08
  out0_bypass : UnitDelay  SampleTime=1e-08
  Q : Outport  SampleTime=1e-08  InitialOutput=0
  wires:
  Trigger_delay_ctrl_const/1 -> Trigger_delay_ctrl_delay/1
  D/1 -> DbypassMux/3
  out0_bypass/1 -> DbypassMux/2
  Trigger_delayed_inverted_and_Trigger/1 -> DbypassMux/1
  Trigger_delay_ctrl_delay/1 -> Trigger_delay_switch/2
  Trigger_delay_Initial_Val/1 -> Trigger_delay_switch/3
  Trigger_delay/1 -> Trigger_delay_switch/1
  not_Trigger_delayed/1 -> Trigger_delayed_inverted_and_Trigger/1
  Trigger_delay_switch/1 -> not_Trigger_delayed/1
  DbypassMux/1 -> out0_bypass/1, Q/1
  Trigger/1 -> Trigger_delay/1, Trigger_delayed_inverted_and_Trigger/2

== system gm_UZ_EnDat_be4_segregation/UZ_ENDAT/CLKDIV7/Triggered Subsystem ==
  D : Inport  OutDataTypeStr=boolean  PortDimensions=1  SampleTime=1e-08
  Trigger : Inport  Port=2  OutDataTypeStr=boolean  SampleTime=1e-08
  DbypassMux : MultiPortSwitch  DataPortOrder=Zero-based contiguous  Inputs=2  zeroidx=on  SampleTime=1e-08  SaturateOnIntegerOverflow=off  InputSameDT=off
  Trigger_delay : Delay  DelayLength=double(1)  InitialCondition=0
  Trigger_delay_Initial_Val : Constant  OutDataTypeStr=boolean  SampleTime=1e-08
  Trigger_delay_ctrl_const : Constant  OutDataTypeStr=boolean  SampleTime=1e-08
  Trigger_delay_ctrl_delay : Delay  DelayLength=double(1)  InitialCondition=0
  Trigger_delay_switch : Switch  Criteria=u2 ~= 0  Threshold=double(0)  OutDataTypeStr=boolean  SampleTime=1e-08  SaturateOnIntegerOverflow=off  InputSameDT=off
  Trigger_delayed_inverted_and_Trigger : Logic  AllPortsSameDT=off  OutDataTypeStr=boolean  SampleTime=1e-08
  not_Trigger_delayed : Logic  Operator=NOT  Inputs=1  AllPortsSameDT=off  OutDataTypeStr=boolean  SampleTime=1e-08
  out0_bypass : UnitDelay  SampleTime=1e-08
  Q : Outport  SampleTime=1e-08  InitialOutput=0
  wires:
  Trigger_delay_ctrl_const/1 -> Trigger_delay_ctrl_delay/1
  D/1 -> DbypassMux/3
  out0_bypass/1 -> DbypassMux/2
  Trigger_delayed_inverted_and_Trigger/1 -> DbypassMux/1
  Trigger_delay_ctrl_delay/1 -> Trigger_delay_switch/2
  Trigger_delay_Initial_Val/1 -> Trigger_delay_switch/3
  Trigger_delay/1 -> Trigger_delay_switch/1
  not_Trigger_delayed/1 -> Trigger_delayed_inverted_and_Trigger/1
  Trigger_delay_switch/1 -> not_Trigger_delayed/1
  DbypassMux/1 -> out0_bypass/1, Q/1
  Trigger/1 -> Trigger_delay/1, Trigger_delayed_inverted_and_Trigger/2

== system gm_UZ_EnDat_be4_segregation/UZ_ENDAT/CLKDIV8/Triggered Subsystem ==
  D : Inport  OutDataTypeStr=boolean  PortDimensions=1  SampleTime=1e-08
  Trigger : Inport  Port=2  OutDataTypeStr=boolean  SampleTime=1e-08
  DbypassMux : MultiPortSwitch  DataPortOrder=Zero-based contiguous  Inputs=2  zeroidx=on  SampleTime=1e-08  SaturateOnIntegerOverflow=off  InputSameDT=off
  Trigger_delay : Delay  DelayLength=double(1)  InitialCondition=0
  Trigger_delay_Initial_Val : Constant  OutDataTypeStr=boolean  SampleTime=1e-08
  Trigger_delay_ctrl_const : Constant  OutDataTypeStr=boolean  SampleTime=1e-08
  Trigger_delay_ctrl_delay : Delay  DelayLength=double(1)  InitialCondition=0
  Trigger_delay_switch : Switch  Criteria=u2 ~= 0  Threshold=double(0)  OutDataTypeStr=boolean  SampleTime=1e-08  SaturateOnIntegerOverflow=off  InputSameDT=off
  Trigger_delayed_inverted_and_Trigger : Logic  AllPortsSameDT=off  OutDataTypeStr=boolean  SampleTime=1e-08
  not_Trigger_delayed : Logic  Operator=NOT  Inputs=1  AllPortsSameDT=off  OutDataTypeStr=boolean  SampleTime=1e-08
  out0_bypass : UnitDelay  SampleTime=1e-08
  Q : Outport  SampleTime=1e-08  InitialOutput=0
  wires:
  Trigger_delay_ctrl_const/1 -> Trigger_delay_ctrl_delay/1
  D/1 -> DbypassMux/3
  out0_bypass/1 -> DbypassMux/2
  Trigger_delayed_inverted_and_Trigger/1 -> DbypassMux/1
  Trigger_delay_ctrl_delay/1 -> Trigger_delay_switch/2
  Trigger_delay_Initial_Val/1 -> Trigger_delay_switch/3
  Trigger_delay/1 -> Trigger_delay_switch/1
  not_Trigger_delayed/1 -> Trigger_delayed_inverted_and_Trigger/1
  Trigger_delay_switch/1 -> not_Trigger_delayed/1
  DbypassMux/1 -> out0_bypass/1, Q/1
  Trigger/1 -> Trigger_delay/1, Trigger_delayed_inverted_and_Trigger/2

== system gm_UZ_EnDat_be4_segregation/UZ_ENDAT/CLKDIV9/Triggered Subsystem ==
  D : Inport  OutDataTypeStr=boolean  PortDimensions=1  SampleTime=1e-08
  Trigger : Inport  Port=2  OutDataTypeStr=boolean  SampleTime=1e-08
  DbypassMux : MultiPortSwitch  DataPortOrder=Zero-based contiguous  Inputs=2  zeroidx=on  SampleTime=1e-08  SaturateOnIntegerOverflow=off  InputSameDT=off
  Trigger_delay : Delay  DelayLength=double(1)  InitialCondition=0
  Trigger_delay_Initial_Val : Constant  OutDataTypeStr=boolean  SampleTime=1e-08
  Trigger_delay_ctrl_const : Constant  OutDataTypeStr=boolean  SampleTime=1e-08
  Trigger_delay_ctrl_delay : Delay  DelayLength=double(1)  InitialCondition=0
  Trigger_delay_switch : Switch  Criteria=u2 ~= 0  Threshold=double(0)  OutDataTypeStr=boolean  SampleTime=1e-08  SaturateOnIntegerOverflow=off  InputSameDT=off
  Trigger_delayed_inverted_and_Trigger : Logic  AllPortsSameDT=off  OutDataTypeStr=boolean  SampleTime=1e-08
  not_Trigger_delayed : Logic  Operator=NOT  Inputs=1  AllPortsSameDT=off  OutDataTypeStr=boolean  SampleTime=1e-08
  out0_bypass : UnitDelay  SampleTime=1e-08
  Q : Outport  SampleTime=1e-08  InitialOutput=0
  wires:
  Trigger_delay_ctrl_const/1 -> Trigger_delay_ctrl_delay/1
  D/1 -> DbypassMux/3
  out0_bypass/1 -> DbypassMux/2
  Trigger_delayed_inverted_and_Trigger/1 -> DbypassMux/1
  Trigger_delay_ctrl_delay/1 -> Trigger_delay_switch/2
  Trigger_delay_Initial_Val/1 -> Trigger_delay_switch/3
  Trigger_delay/1 -> Trigger_delay_switch/1
  not_Trigger_delayed/1 -> Trigger_delayed_inverted_and_Trigger/1
  Trigger_delay_switch/1 -> not_Trigger_delayed/1
  DbypassMux/1 -> out0_bypass/1, Q/1
  Trigger/1 -> Trigger_delay/1, Trigger_delayed_inverted_and_Trigger/2

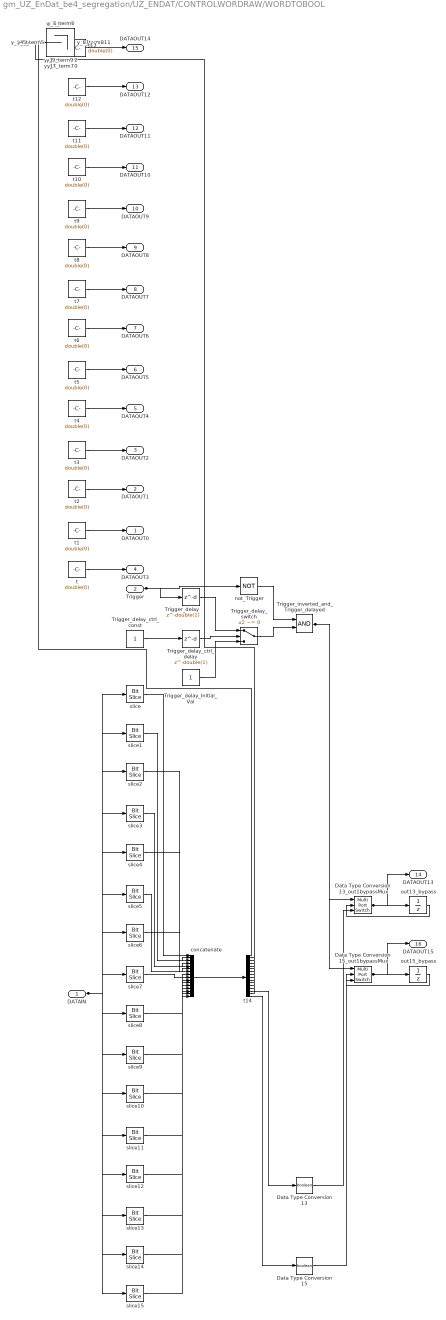
== system gm_UZ_EnDat_be4_segregation/UZ_ENDAT/CONTROLWORDRAW/WORDTOBOOL ==
  DATAIN : Inport  OutDataTypeStr=uint16  PortDimensions=1  SampleTime=1e-08
  Trigger : Inport  Port=2  OutDataTypeStr=boolean  SampleTime=1e-08
  Data Type Conversion13 : DataTypeConversion  OutDataTypeStr=boolean  SampleTime=1e-08  SaturateOnIntegerOverflow=off  RndMeth=Floor
  Data Type Conversion13_out1bypassMux : MultiPortSwitch  DataPortOrder=Zero-based contiguous  Inputs=2  zeroidx=on  SampleTime=1e-08  SaturateOnIntegerOverflow=off  InputSameDT=off
  Data Type Conversion15 : DataTypeConversion  OutDataTypeStr=boolean  SampleTime=1e-08  SaturateOnIntegerOverflow=off  RndMeth=Floor
  Data Type Conversion15_out1bypassMux : MultiPortSwitch  DataPortOrder=Zero-based contiguous  Inputs=2  zeroidx=on  SampleTime=1e-08  SaturateOnIntegerOverflow=off  InputSameDT=off
  Trigger_delay : Delay  DelayLength=double(1)  InitialCondition=0
  Trigger_delay_Initial_Val : Constant  OutDataTypeStr=boolean  SampleTime=1e-08
  Trigger_delay_ctrl_const : Constant  OutDataTypeStr=boolean  SampleTime=1e-08
  Trigger_delay_ctrl_delay : Delay  DelayLength=double(1)  InitialCondition=0
  Trigger_delay_switch : Switch  Criteria=u2 ~= 0  Threshold=double(0)  OutDataTypeStr=boolean  SampleTime=1e-08  SaturateOnIntegerOverflow=off  InputSameDT=off
  Trigger_inverted_and_Trigger_delayed : Logic  AllPortsSameDT=off  OutDataTypeStr=boolean  SampleTime=1e-08
  concatenate : Concatenate  NumInputs=16  Mode=Multidimensional array  ConcatenateDimension=2
  not_Trigger : Logic  Operator=NOT  Inputs=1  AllPortsSameDT=off  OutDataTypeStr=boolean  SampleTime=1e-08
  out13_bypass : UnitDelay  SampleTime=1e-08
  out15_bypass : UnitDelay  SampleTime=1e-08
  slice : hdlsllib/Logic and Bit Operations/Bit Slice  lidx=double(0)  ridx=double(0)
  slice1 : hdlsllib/Logic and Bit Operations/Bit Slice  lidx=double(1)  ridx=double(1)
  slice10 : hdlsllib/Logic and Bit Operations/Bit Slice  lidx=double(10)  ridx=double(10)
  slice11 : hdlsllib/Logic and Bit Operations/Bit Slice  lidx=double(11)  ridx=double(11)
  slice12 : hdlsllib/Logic and Bit Operations/Bit Slice  lidx=double(12)  ridx=double(12)
  slice13 : hdlsllib/Logic and Bit Operations/Bit Slice  lidx=double(13)  ridx=double(13)
  slice14 : hdlsllib/Logic and Bit Operations/Bit Slice  lidx=double(14)  ridx=double(14)
  slice15 : hdlsllib/Logic and Bit Operations/Bit Slice  lidx=double(15)  ridx=double(15)
  slice2 : hdlsllib/Logic and Bit Operations/Bit Slice  lidx=double(2)  ridx=double(2)
  slice3 : hdlsllib/Logic and Bit Operations/Bit Slice  lidx=double(3)  ridx=double(3)
  slice4 : hdlsllib/Logic and Bit Operations/Bit Slice  lidx=double(4)  ridx=double(4)
  slice5 : hdlsllib/Logic and Bit Operations/Bit Slice  lidx=double(5)  ridx=double(5)
  slice6 : hdlsllib/Logic and Bit Operations/Bit Slice  lidx=double(6)  ridx=double(6)
  slice7 : hdlsllib/Logic and Bit Operations/Bit Slice  lidx=double(7)  ridx=double(7)
  slice8 : hdlsllib/Logic and Bit Operations/Bit Slice  lidx=double(8)  ridx=double(8)
  slice9 : hdlsllib/Logic and Bit Operations/Bit Slice  lidx=double(9)  ridx=double(9)
  t{,1..13} (14 alike) : Constant  Value=double(0)  OutDataTypeStr=boolean  SampleTime=1e-08
  t14 : Demux  Outputs=16
  y_0_term0 : Terminator
  y_10_term10 : Terminator
  y_11_term11 : Terminator
  y_12_term12 : Terminator
  y_14_term14 : Terminator
  y_1_term1 : Terminator
  y_2_term2 : Terminator
  y_3_term3 : Terminator
  y_4_term4 : Terminator
  y_5_term5 : Terminator
  y_6_term6 : Terminator
  y_7_term7 : Terminator
  y_8_term8 : Terminator
  y_9_term9 : Terminator
  DATAOUT0 : Outport  SampleTime=1e-08  InitialOutput=0
  DATAOUT1 : Outport  Port=2  SampleTime=1e-08  InitialOutput=0
  DATAOUT2 : Outport  Port=3  SampleTime=1e-08  InitialOutput=0
  DATAOUT3 : Outport  Port=4  SampleTime=1e-08  InitialOutput=0
  DATAOUT4 : Outport  Port=5  SampleTime=1e-08  InitialOutput=0
  DATAOUT5 : Outport  Port=6  SampleTime=1e-08  InitialOutput=0
  DATAOUT6 : Outport  Port=7  SampleTime=1e-08  InitialOutput=0
  DATAOUT7 : Outport  Port=8  SampleTime=1e-08  InitialOutput=0
  DATAOUT8 : Outport  Port=9  SampleTime=1e-08  InitialOutput=0
  DATAOUT9 : Outport  Port=10  SampleTime=1e-08  InitialOutput=0
  DATAOUT10 : Outport  Port=11  SampleTime=1e-08  InitialOutput=0
  DATAOUT11 : Outport  Port=12  SampleTime=1e-08  InitialOutput=0
  DATAOUT12 : Outport  Port=13  SampleTime=1e-08  InitialOutput=0
  DATAOUT13 : Outport  Port=14  SampleTime=1e-08  InitialOutput=0
  DATAOUT14 : Outport  Port=15  SampleTime=1e-08  InitialOutput=0
  DATAOUT15 : Outport  Port=16  SampleTime=1e-08  InitialOutput=0
  wires:
  Trigger/1 -> not_Trigger/1, Trigger_delay/1
  DATAIN/1 -> slice15/1, slice14/1, slice13/1, slice12/1, slice11/1, slice10/1, slice9/1, slice8/1, slice7/1, slice6/1, slice5/1, slice4/1, slice3/1, slice2/1, slice1/1, slice/1
  t1/1 -> DATAOUT0/1
  t2/1 -> DATAOUT1/1
  t3/1 -> DATAOUT2/1
  t/1 -> DATAOUT3/1
  t4/1 -> DATAOUT4/1
  t5/1 -> DATAOUT5/1
  t6/1 -> DATAOUT6/1
  t7/1 -> DATAOUT7/1
  t8/1 -> DATAOUT8/1
  t9/1 -> DATAOUT9/1
  t10/1 -> DATAOUT10/1
  t11/1 -> DATAOUT11/1
  t12/1 -> DATAOUT12/1
  Data Type Conversion13_out1bypassMux/1 -> DATAOUT13/1, out13_bypass/1
  t13/1 -> DATAOUT14/1
  Data Type Conversion15_out1bypassMux/1 -> DATAOUT15/1, out15_bypass/1
  Trigger_delay_switch/1 -> Trigger_inverted_and_Trigger_delayed/2
  not_Trigger/1 -> Trigger_inverted_and_Trigger_delayed/1
  Trigger_inverted_and_Trigger_delayed/1 -> Data Type Conversion13_out1bypassMux/1, Data Type Conversion15_out1bypassMux/1
  Trigger_delay/1 -> Trigger_delay_switch/1
  Trigger_delay_Initial_Val/1 -> Trigger_delay_switch/3
  Trigger_delay_ctrl_const/1 -> Trigger_delay_ctrl_delay/1
  Trigger_delay_ctrl_delay/1 -> Trigger_delay_switch/2
  concatenate/1 -> t14/1
  t14/1 -> y_0_term0/1
  t14/2 -> y_1_term1/1
  t14/3 -> y_2_term2/1
  t14/4 -> y_3_term3/1
  t14/5 -> y_4_term4/1
  t14/6 -> y_5_term5/1
  t14/7 -> y_6_term6/1
  t14/8 -> y_7_term7/1
  t14/9 -> y_8_term8/1
  t14/10 -> y_9_term9/1
  t14/11 -> y_10_term10/1
  t14/12 -> y_11_term11/1
  t14/13 -> y_12_term12/1
  t14/14 -> Data Type Conversion13/1
  t14/15 -> y_14_term14/1
  t14/16 -> Data Type Conversion15/1
  slice/1 -> concatenate/1
  slice1/1 -> concatenate/2
  slice2/1 -> concatenate/3
  slice3/1 -> concatenate/4
  slice4/1 -> concatenate/5
  slice5/1 -> concatenate/6
  slice6/1 -> concatenate/7
  slice7/1 -> concatenate/8
  slice8/1 -> concatenate/9
  slice9/1 -> concatenate/10
  slice10/1 -> concatenate/11
  slice11/1 -> concatenate/12
  slice12/1 -> concatenate/13
  slice13/1 -> concatenate/14
  slice14/1 -> concatenate/15
  slice15/1 -> concatenate/16
  out13_bypass/1 -> Data Type Conversion13_out1bypassMux/2
  Data Type Conversion13/1 -> Data Type Conversion13_out1bypassMux/3
  out15_bypass/1 -> Data Type Conversion15_out1bypassMux/2
  Data Type Conversion15/1 -> Data Type Conversion15_out1bypassMux/3
